simulink model "MIMO_KALMAN_SIMULINK"  (R2026a)
settings: Solver=ode1  StopTime=90.0  FixedStep=0.05
values from neighbouring files (symbols this model uses):
  Aol = sys_d.A    [MIMO_KALMAN_FILTER.m]
  Bol = sys_d.B    [MIMO_KALMAN_FILTER.m]
  Col = sys_d.C    [MIMO_KALMAN_FILTER.m]
undefined symbols (not defined in the file or in its folder): L
libraries: simulink x2
settings Model: Creator=natea  LastModifiedBy=natea

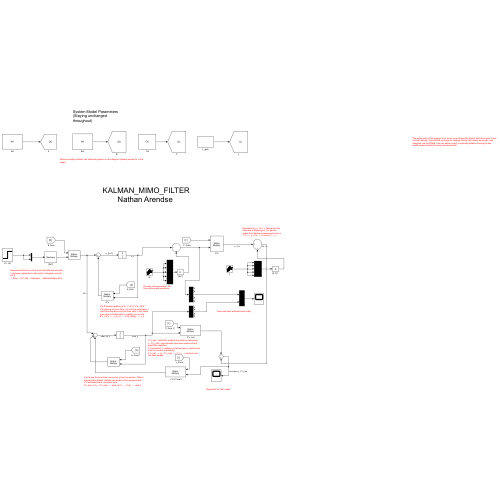
[thumbnail: Simulink's stored preview of the top-level diagram]
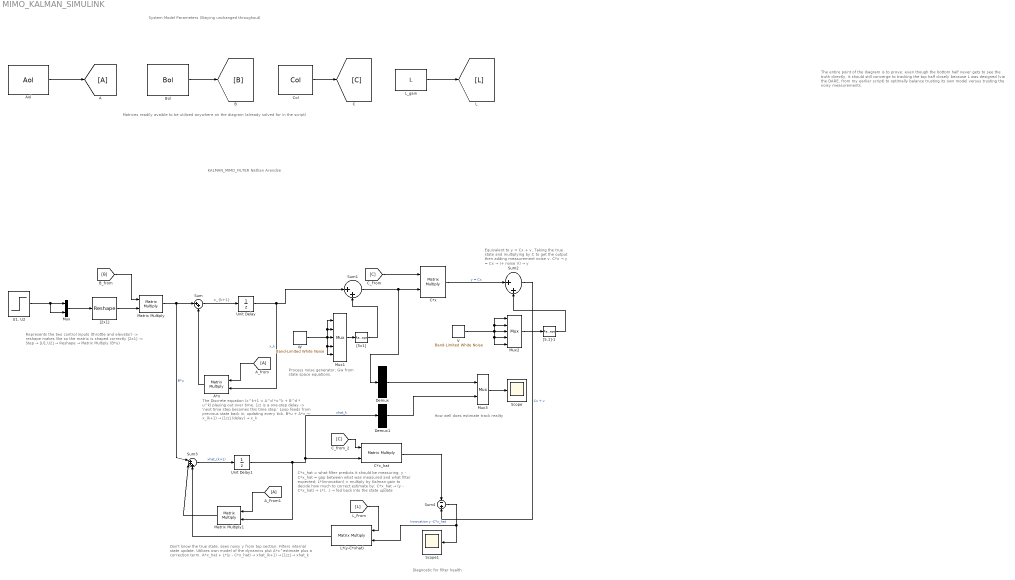
== system MIMO_KALMAN_SIMULINK ==
  note: The entire point of the diagram is to prove: even though the bottom half never gets to see the truth directly, it should still converge to tracking the top half closely because L was designed (via the DARE, from my earlier script) to optimally balance trusting its own model versus trusting the noisy measurements.
  note: How well does estimate track reality
  note: Diagnostic for filter health
  note: C*x_hat = what filter predicts it should be measuring;
      | y - C*x_hat = gap between what was measured and what filter expected;
      | L*(innovation) = multiply by Kalman gain to decide how much to correct estimate by;
      | C*x_hat → (y - C*x_hat) → L*(...) → fed back into the state update
  note: Don't know the true state, sees noisy y from top section. Filters internal state update. Utilizes own model of the dynamics plut A*x^estimate plus a correction term.
      | A*x_hat + L*(y - C*x_hat) → xhat_(k+1) → [1/z] → xhat_k
  note: Equivalent to y = Cx + v. Taking the true state and multiplying by C to get the output then adding measurement noise v.
      | C*x → y = Cx → (+ noise V) → y
  note: Process noise generator; Gw from state space equations.
  note: The Discrete equation (x^k+1 = A^d *x^k + B^d * u^k) playing out over time. 1/z is a one-step delay -> 'next time step becomes this time step.' Loop feeds from previous state back in, updating every tick.
      | B*u + A*x → x_(k+1) → [1/z] (delay) → x_k
  note: Represents the two control inputs (throttle and elevator) -> reshape makes like so the matrix is shaped correctly [2x1]
      | -> Step → [U1,U2] → Reshape → Matrix Multiply (B*u)
  note: Matrices readily avaible to be utilized anywhere on the diagram (already solved for in the script)
  note: KALMAN_MIMO_FILTER
      | Nathan Arendse
  note: x_{k+1}
  note: System Model Parameters (Staying unchanged throughout)
  A : Goto
  A*x : Product  Multiplication=Matrix(*)
  A_From1 : From
  A_from : From
  Aol : Constant  Value=Aol
  Bol : Constant  Value=Bol
  C*x : Product  Multiplication=Matrix(*)
  C*x_hat : Product  Multiplication=Matrix(*)
  Col : Constant  Value=Col
  Demux : Demux  Outputs=5
  Demux1 : Demux  Outputs=5
  L*(y-C*xhat) : Product  Multiplication=Matrix(*)
  L_gain : Constant  Value=L
  Matrix Multiply : Product  Multiplication=Matrix(*)
  Matrix Multiply1 : Product  Multiplication=Matrix(*)
  Mux : Mux  Inputs=2
  Mux1 : Mux  Inputs=5
  Mux2 : Mux  Inputs=5
  Mux3 : Mux  Inputs=2
  Scope : Scope
      settings: Title=True Output vs. Kalman Filter Estimate  ActiveDisplayYMinimum=-2.96664637434703  ActiveDisplayYMaximum=-2.7506428959480962  YLabel=Output/State Value
  Scope1 : Scope
      settings: ActiveDisplayYMinimum=-40.943828324500316  ActiveDisplayYMaximum=36.528685499097669
  Sum : Sum  Inputs=|++
  Sum1 : Sum  Inputs=|++
  Sum2 : Sum  Inputs=|++
  Sum3 : Sum  Inputs=|+++
  Sum4 : Sum  Inputs=-+
  "U1, U2" : Step  SampleTime=0
  Unit Delay : UnitDelay  SampleTime=-1
  Unit Delay1 : UnitDelay  SampleTime=-1
  V : simulink/Sources/Band-Limited White Noise  Cov=[0.1]  Ts=0.05  seed=[23341]
  W : simulink/Sources/Band-Limited White Noise  Cov=[0.1]  Ts=0.05  seed=[23341]
  "[2x1]" : Reshape  OutputDimensionality=Customize  OutputDimensions=[2,1]
  "[5,1]-1" : Reshape  OutputDimensionality=Customize  OutputDimensions=[5,1]
  "[5x1]" : Reshape  OutputDimensionality=Customize  OutputDimensions=[5,1]
  wires:
  Aol/1 -> A/1
  Bol/1 -> [B]
  Col/1 -> [C]
  L_gain/1 -> [L]
  [B] -> Matrix Multiply/1
  "[2x1]"/1 -> Matrix Multiply/2
  Matrix Multiply/1 -> Sum3/1, Sum/1  "B*u"
  "U1, U2"/1 -> Mux/2, Mux/1
  Mux/1 -> "[2x1]"/1
  Sum/1 -> Unit Delay/1
  Unit Delay/1 -> Sum1/1, A*x/2  "x_k"
  A_from/1 -> A*x/1
  A*x/1 -> Sum/2
  W/1 -> Mux1/5, Mux1/4, Mux1/1, Mux1/2, Mux1/3
  Mux1/1 -> "[5x1]"/1
  "[5x1]"/1 -> Sum1/2
  Sum1/1 -> Demux/1, C*x/2
  [C] -> C*x/1
  C*x/1 -> Sum2/1  "y = Cx"
  V/1 -> Mux2/5, Mux2/4, Mux2/1, Mux2/2, Mux2/3
  Mux2/1 -> "[5,1]-1"/1
  "[5,1]-1"/1 -> Sum2/2
  Sum2/1 -> Sum4/2  "Cx + v"
  Sum3/1 -> Unit Delay1/1  "xhat_(k+1)"
  Matrix Multiply1/1 -> Sum3/2
  A_From1/1 -> Matrix Multiply1/1
  Unit Delay1/1 -> Matrix Multiply1/2, Demux1/1, C*x_hat/2  "xhat_k"
  [C] -> C*x_hat/1
  C*x_hat/1 -> Sum4/1
  Sum4/1 -> Scope1/1, L*(y-C*xhat)/2  "Innovation y -C*x_hat"
  [L] -> L*(y-C*xhat)/1
  L*(y-C*xhat)/1 -> Sum3/3
  Mux3/1 -> Scope/1
  Demux/3 -> Mux3/1
  Demux1/3 -> Mux3/2
